simulink model "Simulink_deliverable_2"  (R2025b)
settings: Solver=VariableStepAuto  StartTime=0.0  StopTime=10.0  RelTol=1e-3
settings Model: Creator=20233602  LastModifiedBy=20233602

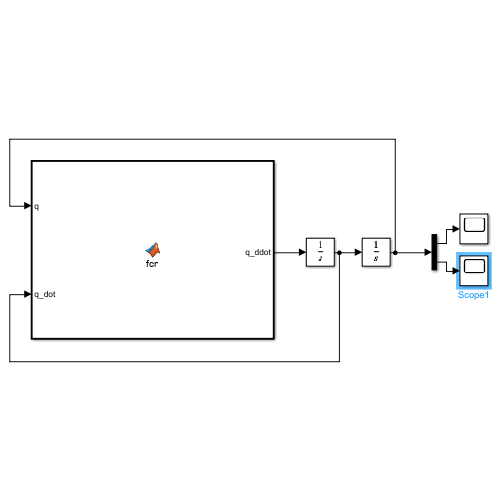
[thumbnail: Simulink's stored preview of the top-level diagram]
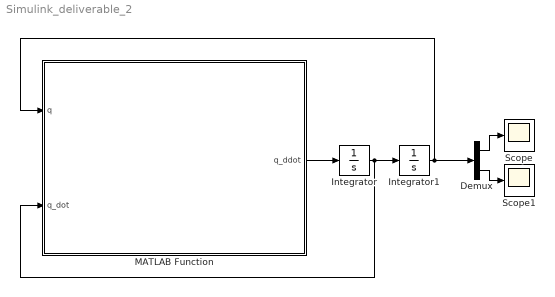
== system Simulink_deliverable_2 ==
  Demux : Demux  Outputs=2
  Integrator : Integrator  InitialCondition=[0,0]
  Integrator1 : Integrator  InitialCondition=[11.5, pi/3]
  MATLAB Function : MATLAB Function  TreatAsAtomicUnit=on
  Scope : Scope
      settings: ActiveDisplayYMinimum=11.322925454107702  ActiveDisplayYMaximum=13.093670913030691
  Scope1 : Scope
      settings: ActiveDisplayYMinimum=0.937355315626571  ActiveDisplayYMaximum=2.0357776713268381
  wires:
  MATLAB Function/1(q_ddot) -> Integrator/1
  Integrator/1 -> MATLAB Function/2(q_dot), Integrator1/1
  Integrator1/1 -> MATLAB Function/1(q), Demux/1
  Demux/1 -> Scope/1
  Demux/2 -> Scope1/1

== matlab function Simulink_deliverable_2/MATLAB Function ==
  data: q_ddot output; q input; q_dot input
function q_ddot = fcn(q,q_dot)

%Generalized constants
x = q(1);
theta = q(2);
x_dot = q_dot(1);
theta_dot = q_dot(2);

%M and F
M = [2500, 5000*sin(391/250);
     5000*sin(391/250), 50000];

F = [-7000*x - 200*x_dot - 2000*sin(391/250)*theta_dot + 87500;
     -20010*theta_dot - (49050*sin(391/250) + 200)*(theta - 391/250)];

q_ddot= transpose(M\F);
